simulink model "Bug_LibraryBlock&StateWriter"  (R2020b)
settings: Solver=VariableStepAuto  StartTime=0.0  StopTime=10.0  RelTol=1e-3
undefined symbols (not defined in the file): DiscIntNeverNeededParam
settings Model: Creator=alons  LastModifiedBy=alons

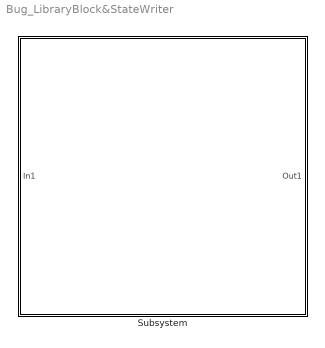
== system Bug_LibraryBlock&StateWriter ==
  Subsystem : Subsystem  Variant=on  VariantControlMode=label  VariantControl=Choice  LabelModeActiveChoice=Choice2

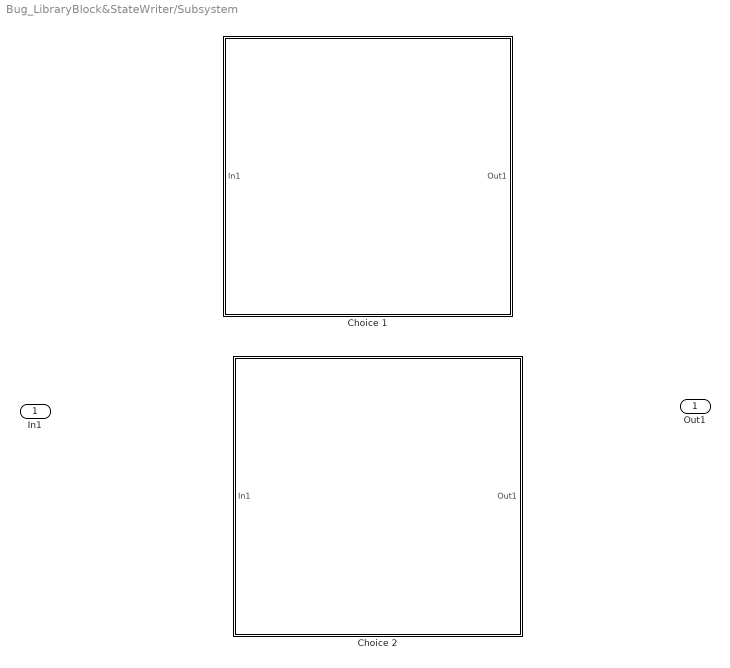
== system Bug_LibraryBlock&StateWriter/Subsystem ==
  In1 : Inport
  Choice 1 : Subsystem  VariantControl=Choice1
  Choice 2 : Subsystem  VariantControl=Choice2
  Out1 : Outport

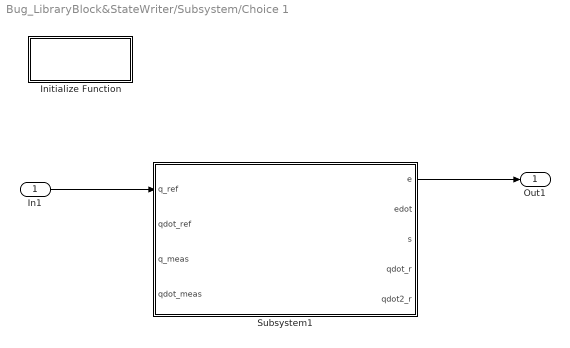
== system Bug_LibraryBlock&StateWriter/Subsystem/Choice 1 ==
  In1 : Inport
  Initialize Function : Subsystem  TreatAsAtomicUnit=on
  Subsystem1 : Subsystem
  Out1 : Outport
  wires:
  In1/1 -> Subsystem1/1(q_ref)
  Subsystem1/1(e) -> Out1/1

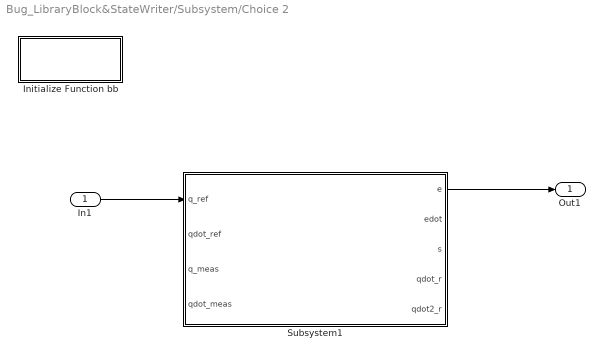
== system Bug_LibraryBlock&StateWriter/Subsystem/Choice 2 ==
  In1 : Inport
  Initialize Function bb : Subsystem  TreatAsAtomicUnit=on
  Subsystem1 : Subsystem
  Out1 : Outport
  wires:
  In1/1 -> Subsystem1/1(q_ref)
  Subsystem1/1(e) -> Out1/1

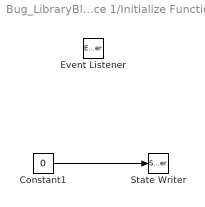
== system Bug_LibraryBlock&StateWriter/Subsystem/Choice 1/Initialize Function ==
  Constant1 : Constant  Value=0
  Event Listener : EventListener  DisableCoverage=on  EventName=reset
  State Writer : StateWriter  StateOwnerBlock=../../Subsystem1/LPF/Discrete-Time Integrator1
  wires:
  Constant1/1 -> State Writer/1

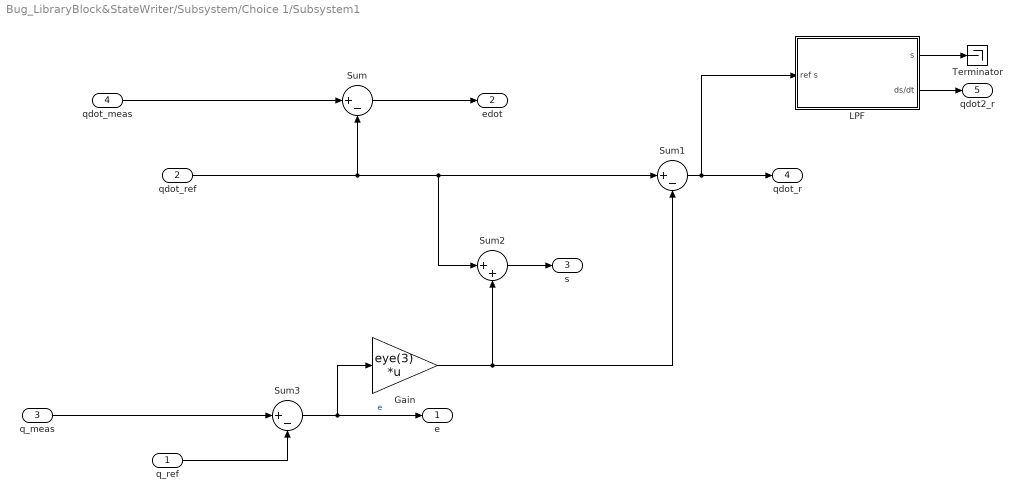
== system Bug_LibraryBlock&StateWriter/Subsystem/Choice 1/Subsystem1 ==
  q_ref : Inport  PortDimensions=3
  qdot_ref : Inport  Port=2  PortDimensions=3
  q_meas : Inport  Port=3  PortDimensions=3
  qdot_meas : Inport  Port=4  PortDimensions=3
  Gain : Gain  Gain=eye(3)  Multiplication=Matrix(K*u) (u vector)
  LPF : Subsystem  mask{Freq=100, s0=0}
      mask prompts: Freq "LPF Freq [Hz]"
      mask Display: fprintf('LPF %g[Hz]',Freq);
  Sum : Sum  Inputs=|+-
  Sum1 : Sum  Inputs=|+-
  Sum2 : Sum  Inputs=|++
  Sum3 : Sum  Inputs=|+-
  Terminator : Terminator
  e : Outport  PortDimensions=3
  edot : Outport  Port=2  PortDimensions=3
  s : Outport  Port=3  PortDimensions=3
  qdot_r : Outport  Port=4  PortDimensions=3
  qdot2_r : Outport  Port=5  PortDimensions=3
  wires:
  qdot_meas/1 -> Sum/1
  qdot_ref/1 -> Sum2/1, Sum1/1, Sum/2
  Sum/1 -> edot/1
  Sum2/1 -> s/1
  q_ref/1 -> Sum3/2
  q_meas/1 -> Sum3/1
  Gain/1 -> Sum2/2, Sum1/2
  Sum1/1 -> LPF/1(ref s), qdot_r/1
  LPF/1(s) -> Terminator/1
  LPF/2(ds/dt) -> qdot2_r/1
  Sum3/1 -> Gain/1, e/1  "e"

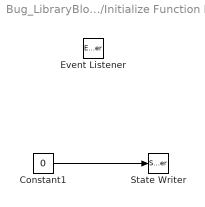
== system Bug_LibraryBlock&StateWriter/Subsystem/Choice 2/Initialize Function bb ==
  Constant1 : Constant  Value=0
  Event Listener : EventListener  DisableCoverage=on  EventName=reset
  State Writer : StateWriter  StateOwnerBlock=../../Subsystem1/LPF/Discrete-Time Integrator1
  wires:
  Constant1/1 -> State Writer/1

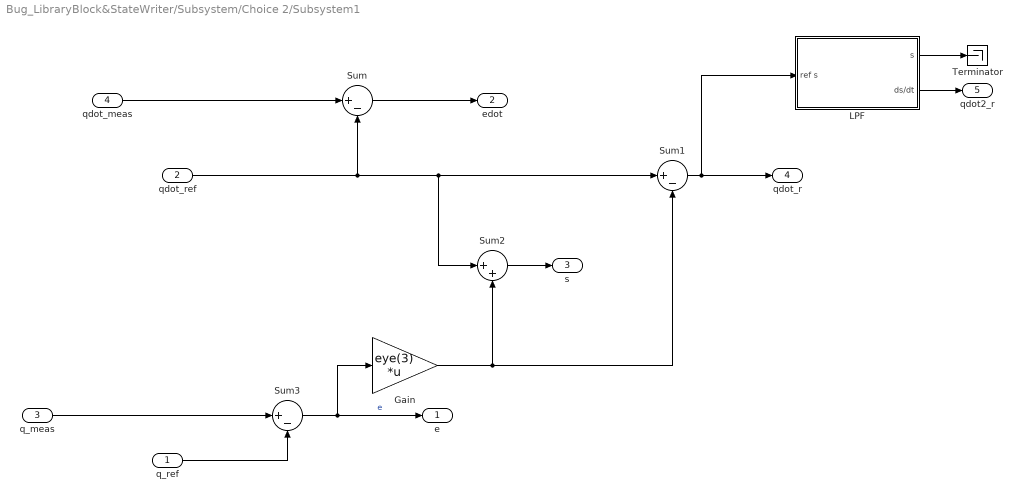
== system Bug_LibraryBlock&StateWriter/Subsystem/Choice 2/Subsystem1 ==
  q_ref : Inport  PortDimensions=3
  qdot_ref : Inport  Port=2  PortDimensions=3
  q_meas : Inport  Port=3  PortDimensions=3
  qdot_meas : Inport  Port=4  PortDimensions=3
  Gain : Gain  Gain=eye(3)  Multiplication=Matrix(K*u) (u vector)
  LPF : Subsystem  mask{Freq=100, s0=0}
      mask prompts: Freq "LPF Freq [Hz]"
      mask Display: fprintf('LPF %g[Hz]',Freq);
  Sum : Sum  Inputs=|+-
  Sum1 : Sum  Inputs=|+-
  Sum2 : Sum  Inputs=|++
  Sum3 : Sum  Inputs=|+-
  Terminator : Terminator
  e : Outport  PortDimensions=3
  edot : Outport  Port=2  PortDimensions=3
  s : Outport  Port=3  PortDimensions=3
  qdot_r : Outport  Port=4  PortDimensions=3
  qdot2_r : Outport  Port=5  PortDimensions=3
  wires:
  qdot_meas/1 -> Sum/1
  qdot_ref/1 -> Sum2/1, Sum1/1, Sum/2
  Sum/1 -> edot/1
  Sum2/1 -> s/1
  q_ref/1 -> Sum3/2
  q_meas/1 -> Sum3/1
  Gain/1 -> Sum2/2, Sum1/2
  Sum1/1 -> LPF/1(ref s), qdot_r/1
  LPF/1(s) -> Terminator/1
  LPF/2(ds/dt) -> qdot2_r/1
  Sum3/1 -> Gain/1, e/1  "e"

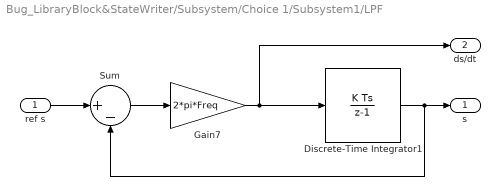
== system Bug_LibraryBlock&StateWriter/Subsystem/Choice 1/Subsystem1/LPF ==
  ref s : Inport
  Discrete-Time Integrator1 : DiscreteIntegrator  InitialCondition=s0  SampleTime=-1  ICPrevOutput=DiscIntNeverNeededParam  ICPrevScaledInput=DiscIntNeverNeededParam
  Gain7 : Gain  Gain=2*pi*Freq
  Sum : Sum  Inputs=|+-
  s : Outport  VectorParamsAs1DForOutWhenUnconnected=off
  ds/dt : Outport  Port=2  VectorParamsAs1DForOutWhenUnconnected=off
  wires:
  Gain7/1 -> Discrete-Time Integrator1/1, ds/dt/1
  ref s/1 -> Sum/1
  Sum/1 -> Gain7/1
  Discrete-Time Integrator1/1 -> s/1, Sum/2

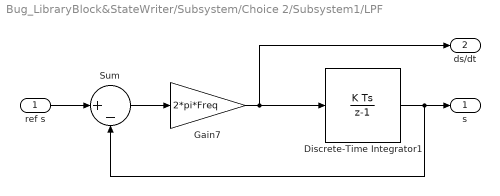
== system Bug_LibraryBlock&StateWriter/Subsystem/Choice 2/Subsystem1/LPF ==
  ref s : Inport
  Discrete-Time Integrator1 : DiscreteIntegrator  InitialCondition=s0  SampleTime=-1  ICPrevOutput=DiscIntNeverNeededParam  ICPrevScaledInput=DiscIntNeverNeededParam
  Gain7 : Gain  Gain=2*pi*Freq
  Sum : Sum  Inputs=|+-
  s : Outport  VectorParamsAs1DForOutWhenUnconnected=off
  ds/dt : Outport  Port=2  VectorParamsAs1DForOutWhenUnconnected=off
  wires:
  Gain7/1 -> Discrete-Time Integrator1/1, ds/dt/1
  ref s/1 -> Sum/1
  Sum/1 -> Gain7/1
  Discrete-Time Integrator1/1 -> s/1, Sum/2
